simulink model "main"  (R2021b)
settings: Solver=ode45  StartTime=0.0  StopTime=15  MaxStep=0.0050000000000000001  RelTol=1.0000000000000001e-09  AbsTol=9.9999999999999994e-12
settings Model: Creator=Lenovo  LastModifiedBy=Lenovo
settings DataIOCC: SaveOutput=off  SignalLogging=off  SaveTime=off  OutputOption=SpecifiedOutputTimes  OutputTimes=0:0.005:15

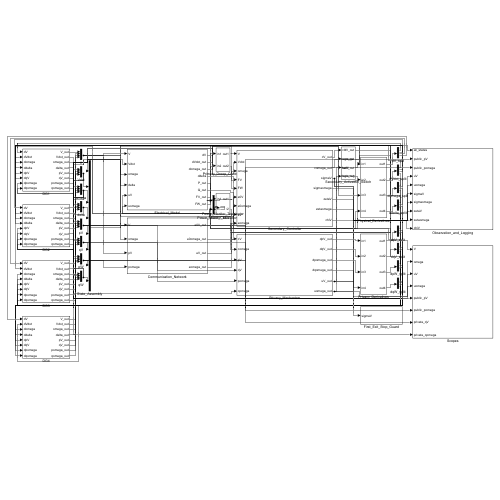
[thumbnail: Simulink's stored preview of the top-level diagram]
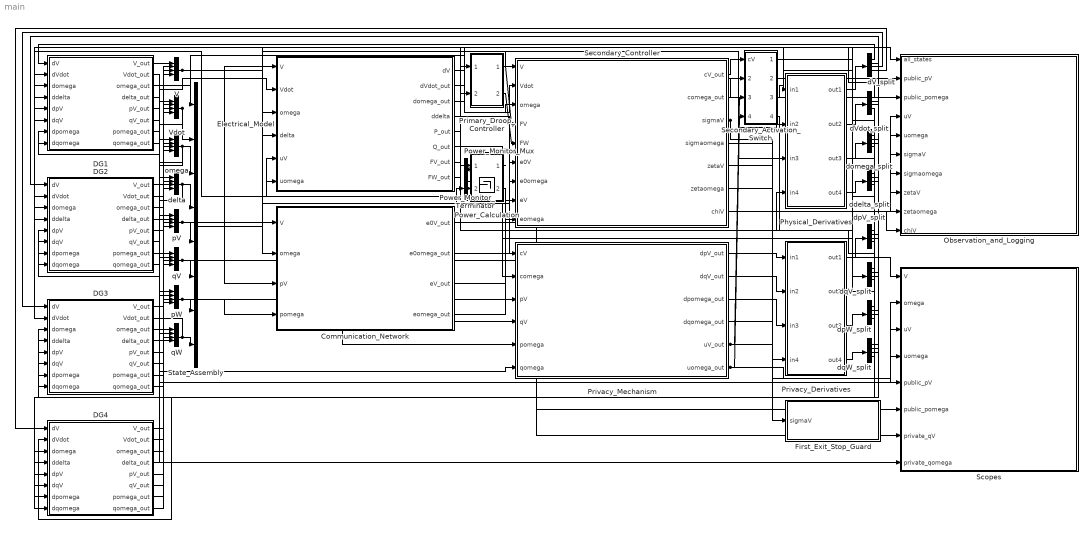
== system main ==
  Communication_Network : Subsystem
  DG1 : Subsystem
  DG2 : Subsystem
  DG3 : Subsystem
  DG4 : Subsystem
  Electrical_Model : Subsystem
  First_Exit_Stop_Guard : Subsystem
  Observation_and_Logging : Subsystem
  Physical_Derivatives : Subsystem
  Power_Calculation : Subsystem
  Power_Monitor_Mux : Mux  Inputs=2
  Power_Monitor_Terminator : Terminator
  Primary_Droop_Controller : Subsystem
  Privacy_Derivatives : Subsystem
  Privacy_Mechanism : Subsystem
  Scopes : Subsystem
  Secondary_Activation_Switch : Subsystem
  Secondary_Controller : Subsystem
  State_Assembly : Mux  Inputs=8
  V : Mux
  Vdot : Mux
  dV_split : Demux
  dVdot_split : Demux
  ddelta_split : Demux
  delta : Mux
  domega_split : Demux
  dpV_split : Demux
  dpW_split : Demux
  dqV_split : Demux
  dqW_split : Demux
  omega : Mux
  pV : Mux
  pW : Mux
  qV : Mux
  qW : Mux
  wires:
  DG1/1(V_out) -> V/1
  DG2/1(V_out) -> V/2
  DG3/1(V_out) -> V/3
  DG4/1(V_out) -> V/4
  V/1 -> State_Assembly/1, Electrical_Model/1(V), Communication_Network/1(V), Secondary_Controller/1(V), Scopes/1(V)
  DG1/2(Vdot_out) -> Vdot/1
  DG2/2(Vdot_out) -> Vdot/2
  DG3/2(Vdot_out) -> Vdot/3
  DG4/2(Vdot_out) -> Vdot/4
  Vdot/1 -> State_Assembly/2, Electrical_Model/2(Vdot), Secondary_Controller/2(Vdot)
  DG1/3(omega_out) -> omega/1
  DG2/3(omega_out) -> omega/2
  DG3/3(omega_out) -> omega/3
  DG4/3(omega_out) -> omega/4
  omega/1 -> State_Assembly/3, Electrical_Model/3(omega), Communication_Network/2(omega), Secondary_Controller/3(omega), Scopes/2(omega)
  DG1/4(delta_out) -> delta/1
  DG2/4(delta_out) -> delta/2
  DG3/4(delta_out) -> delta/3
  DG4/4(delta_out) -> delta/4
  delta/1 -> State_Assembly/4, Electrical_Model/4(delta)
  DG1/5(pV_out) -> pV/1
  DG2/5(pV_out) -> pV/2
  DG3/5(pV_out) -> pV/3
  DG4/5(pV_out) -> pV/4
  pV/1 -> State_Assembly/5, Communication_Network/3(pV), Privacy_Mechanism/3(pV), Observation_and_Logging/2(public_pV), Scopes/5(public_pV)
  DG1/6(qV_out) -> qV/1
  DG2/6(qV_out) -> qV/2
  DG3/6(qV_out) -> qV/3
  DG4/6(qV_out) -> qV/4
  qV/1 -> State_Assembly/6, Privacy_Mechanism/4(qV), Scopes/7(private_qV)
  DG1/7(pomega_out) -> pW/1
  DG2/7(pomega_out) -> pW/2
  DG3/7(pomega_out) -> pW/3
  DG4/7(pomega_out) -> pW/4
  pW/1 -> State_Assembly/7, Communication_Network/4(pomega), Privacy_Mechanism/5(pomega), Observation_and_Logging/3(public_pomega), Scopes/6(public_pomega)
  DG1/8(qomega_out) -> qW/1
  DG2/8(qomega_out) -> qW/2
  DG3/8(qomega_out) -> qW/3
  DG4/8(qomega_out) -> qW/4
  qW/1 -> State_Assembly/8, Privacy_Mechanism/6(qomega), Scopes/8(private_qomega)
  Secondary_Activation_Switch/3(hatV_out) -> Electrical_Model/5(uV)
  Secondary_Activation_Switch/4(hatomega_out) -> Electrical_Model/6(uomega)
  Electrical_Model/1(dV) -> Physical_Derivatives/1(in1)
  Electrical_Model/2(dVdot_out) -> Physical_Derivatives/2(in2)
  Electrical_Model/3(domega_out) -> Physical_Derivatives/3(in3)
  Electrical_Model/4(ddelta) -> Physical_Derivatives/4(in4)
  Electrical_Model/7(FV_out) -> Primary_Droop_Controller/1(in1)
  Electrical_Model/8(FW_out) -> Primary_Droop_Controller/2(in2)
  Primary_Droop_Controller/1(out1) -> Secondary_Controller/4(FV)
  Primary_Droop_Controller/2(out2) -> Secondary_Controller/5(FW)
  Electrical_Model/5(P_out) -> Power_Calculation/1(in1)
  Electrical_Model/6(Q_out) -> Power_Calculation/2(in2)
  Power_Calculation/1(out1) -> Power_Monitor_Mux/1
  Power_Calculation/2(out2) -> Power_Monitor_Mux/2
  Power_Monitor_Mux/1 -> Power_Monitor_Terminator/1
  Communication_Network/1(e0V_out) -> Secondary_Controller/6(e0V)
  Communication_Network/2(e0omega_out) -> Secondary_Controller/7(e0omega)
  Communication_Network/3(eV_out) -> Secondary_Controller/8(eV)
  Communication_Network/4(eomega_out) -> Secondary_Controller/9(eomega)
  Secondary_Controller/1(cV_out) -> Secondary_Activation_Switch/1(cV)
  Secondary_Controller/2(comega_out) -> Secondary_Activation_Switch/2(comega)
  Secondary_Activation_Switch/1(cV_out) -> Privacy_Mechanism/1(cV)
  Secondary_Activation_Switch/2(comega_out) -> Privacy_Mechanism/2(comega)
  Privacy_Mechanism/5(uV_out) -> Secondary_Activation_Switch/3(hatV), Observation_and_Logging/4(uV), Scopes/3(uV)
  Privacy_Mechanism/6(uomega_out) -> Secondary_Activation_Switch/4(hatomega), Observation_and_Logging/5(uomega), Scopes/4(uomega)
  Privacy_Mechanism/1(dpV_out) -> Privacy_Derivatives/1(in1)
  Privacy_Mechanism/2(dqV_out) -> Privacy_Derivatives/2(in2)
  Privacy_Mechanism/3(dpomega_out) -> Privacy_Derivatives/3(in3)
  Privacy_Mechanism/4(dqomega_out) -> Privacy_Derivatives/4(in4)
  Physical_Derivatives/1(out1) -> dV_split/1
  dV_split/1 -> DG1/1(dV)
  dV_split/2 -> DG2/1(dV)
  dV_split/3 -> DG3/1(dV)
  dV_split/4 -> DG4/1(dV)
  Physical_Derivatives/2(out2) -> dVdot_split/1
  dVdot_split/1 -> DG1/2(dVdot)
  dVdot_split/2 -> DG2/2(dVdot)
  dVdot_split/3 -> DG3/2(dVdot)
  dVdot_split/4 -> DG4/2(dVdot)
  Physical_Derivatives/3(out3) -> domega_split/1
  domega_split/1 -> DG1/3(domega)
  domega_split/2 -> DG2/3(domega)
  domega_split/3 -> DG3/3(domega)
  domega_split/4 -> DG4/3(domega)
  Physical_Derivatives/4(out4) -> ddelta_split/1
  ddelta_split/1 -> DG1/4(ddelta)
  ddelta_split/2 -> DG2/4(ddelta)
  ddelta_split/3 -> DG3/4(ddelta)
  ddelta_split/4 -> DG4/4(ddelta)
  Privacy_Derivatives/1(out1) -> dpV_split/1
  dpV_split/1 -> DG1/5(dpV)
  dpV_split/2 -> DG2/5(dpV)
  dpV_split/3 -> DG3/5(dpV)
  dpV_split/4 -> DG4/5(dpV)
  Privacy_Derivatives/2(out2) -> dqV_split/1
  dqV_split/1 -> DG1/6(dqV)
  dqV_split/2 -> DG2/6(dqV)
  dqV_split/3 -> DG3/6(dqV)
  dqV_split/4 -> DG4/6(dqV)
  Privacy_Derivatives/3(out3) -> dpW_split/1
  dpW_split/1 -> DG1/7(dpomega)
  dpW_split/2 -> DG2/7(dpomega)
  dpW_split/3 -> DG3/7(dpomega)
  dpW_split/4 -> DG4/7(dpomega)
  Privacy_Derivatives/4(out4) -> dqW_split/1
  dqW_split/1 -> DG1/8(dqomega)
  dqW_split/2 -> DG2/8(dqomega)
  dqW_split/3 -> DG3/8(dqomega)
  dqW_split/4 -> DG4/8(dqomega)
  State_Assembly/1 -> Observation_and_Logging/1(all_states)
  Secondary_Controller/3(sigmaV) -> Observation_and_Logging/6(sigmaV), First_Exit_Stop_Guard/1(sigmaV)
  Secondary_Controller/4(sigmaomega) -> Observation_and_Logging/7(sigmaomega)
  Secondary_Controller/5(zetaV) -> Observation_and_Logging/8(zetaV)
  Secondary_Controller/6(zetaomega) -> Observation_and_Logging/9(zetaomega)
  Secondary_Controller/7(chiV) -> Observation_and_Logging/10(chiV)

== system main/Communication_Network ==
  V : Inport
  omega : Inport  Port=2
  pV : Inport  Port=3
  pomega : Inport  Port=4
  LpV : Gain  Gain=[1 -1 0 0;-1 2 -1 0;0 -1 2 -1;0 0 -1 1]  Multiplication=Matrix(K*u)
  LpW : Gain  Gain=[1 -1 0 0;-1 2 -1 0;0 -1 2 -1;0 0 -1 1]  Multiplication=Matrix(K*u)
  e0V : Bias  Bias=-1
  e0V_Gain : Gain  Gain=[1 0 0 0;0 1 0 0;0 0 1 0;0 0 0 1]  Multiplication=Matrix(K*u)
  e0omega : Bias
  e0omega_Gain : Gain  Gain=[1 0 0 0;0 1 0 0;0 0 1 0;0 0 0 1]  Multiplication=Matrix(K*u)
  eV : Sum
  eW : Sum
  pinV : Gain  Gain=[1 0 0 0;0 0 0 0;0 0 0 0;0 0 0 0]  Multiplication=Matrix(K*u)
  pinW : Gain  Gain=[1 0 0 0;0 0 0 0;0 0 0 0;0 0 0 0]  Multiplication=Matrix(K*u)
  e0V_out : Outport
  e0omega_out : Outport  Port=2
  eV_out : Outport  Port=3
  eomega_out : Outport  Port=4
  wires:
  V/1 -> e0V/1
  e0V/1 -> e0V_Gain/1
  omega/1 -> e0omega/1
  e0omega/1 -> e0omega_Gain/1
  e0V_Gain/1 -> pinV/1, e0V_out/1
  pV/1 -> LpV/1
  e0omega_Gain/1 -> pinW/1, e0omega_out/1
  pomega/1 -> LpW/1
  pinV/1 -> eV/1
  LpV/1 -> eV/2
  pinW/1 -> eW/1
  LpW/1 -> eW/2
  eV/1 -> eV_out/1
  eW/1 -> eomega_out/1

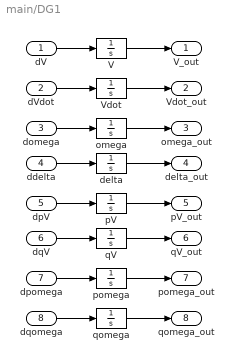
== system main/DG1 ==
  dV : Inport
  dVdot : Inport  Port=2
  domega : Inport  Port=3
  ddelta : Inport  Port=4
  dpV : Inport  Port=5
  dqV : Inport  Port=6
  dpomega : Inport  Port=7
  dqomega : Inport  Port=8
  V : Integrator  InitialCondition=1.0012000000000001
  Vdot : Integrator
  delta : Integrator  InitialCondition=0.01
  omega : Integrator  InitialCondition=0.00069999999999999999
  pV : Integrator  InitialCondition=0.01
  pomega : Integrator  InitialCondition=0.0080000000000000002
  qV : Integrator  InitialCondition=-0.01
  qomega : Integrator  InitialCondition=-0.0080000000000000002
  V_out : Outport
  Vdot_out : Outport  Port=2
  omega_out : Outport  Port=3
  delta_out : Outport  Port=4
  pV_out : Outport  Port=5
  qV_out : Outport  Port=6
  pomega_out : Outport  Port=7
  qomega_out : Outport  Port=8
  wires:
  dV/1 -> V/1
  V/1 -> V_out/1
  dVdot/1 -> Vdot/1
  Vdot/1 -> Vdot_out/1
  domega/1 -> omega/1
  omega/1 -> omega_out/1
  ddelta/1 -> delta/1
  delta/1 -> delta_out/1
  dpV/1 -> pV/1
  pV/1 -> pV_out/1
  dqV/1 -> qV/1
  qV/1 -> qV_out/1
  dpomega/1 -> pomega/1
  pomega/1 -> pomega_out/1
  dqomega/1 -> qomega/1
  qomega/1 -> qomega_out/1

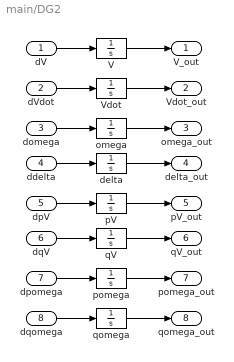
== system main/DG2 ==
  dV : Inport
  dVdot : Inport  Port=2
  domega : Inport  Port=3
  ddelta : Inport  Port=4
  dpV : Inport  Port=5
  dqV : Inport  Port=6
  dpomega : Inport  Port=7
  dqomega : Inport  Port=8
  V : Integrator  InitialCondition=1.0009999999999999
  Vdot : Integrator
  delta : Integrator  InitialCondition=0.0050000000000000001
  omega : Integrator  InitialCondition=0.00050000000000000001
  pV : Integrator  InitialCondition=-0.0080000000000000002
  pomega : Integrator  InitialCondition=-0.0060000000000000001
  qV : Integrator  InitialCondition=0.0080000000000000002
  qomega : Integrator  InitialCondition=0.0060000000000000001
  V_out : Outport
  Vdot_out : Outport  Port=2
  omega_out : Outport  Port=3
  delta_out : Outport  Port=4
  pV_out : Outport  Port=5
  qV_out : Outport  Port=6
  pomega_out : Outport  Port=7
  qomega_out : Outport  Port=8
  wires:
  dV/1 -> V/1
  V/1 -> V_out/1
  dVdot/1 -> Vdot/1
  Vdot/1 -> Vdot_out/1
  domega/1 -> omega/1
  omega/1 -> omega_out/1
  ddelta/1 -> delta/1
  delta/1 -> delta_out/1
  dpV/1 -> pV/1
  pV/1 -> pV_out/1
  dqV/1 -> qV/1
  qV/1 -> qV_out/1
  dpomega/1 -> pomega/1
  pomega/1 -> pomega_out/1
  dqomega/1 -> qomega/1
  qomega/1 -> qomega_out/1

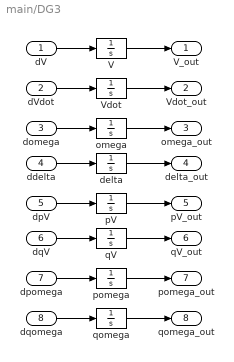
== system main/DG3 ==
  dV : Inport
  dVdot : Inport  Port=2
  domega : Inport  Port=3
  ddelta : Inport  Port=4
  dpV : Inport  Port=5
  dqV : Inport  Port=6
  dpomega : Inport  Port=7
  dqomega : Inport  Port=8
  V : Integrator  InitialCondition=1.0007999999999999
  Vdot : Integrator
  delta : Integrator  InitialCondition=-0.0030000000000000001
  omega : Integrator  InitialCondition=0.00040000000000000002
  pV : Integrator  InitialCondition=0.0060000000000000001
  pomega : Integrator  InitialCondition=0.0050000000000000001
  qV : Integrator  InitialCondition=-0.0060000000000000001
  qomega : Integrator  InitialCondition=-0.0050000000000000001
  V_out : Outport
  Vdot_out : Outport  Port=2
  omega_out : Outport  Port=3
  delta_out : Outport  Port=4
  pV_out : Outport  Port=5
  qV_out : Outport  Port=6
  pomega_out : Outport  Port=7
  qomega_out : Outport  Port=8
  wires:
  dV/1 -> V/1
  V/1 -> V_out/1
  dVdot/1 -> Vdot/1
  Vdot/1 -> Vdot_out/1
  domega/1 -> omega/1
  omega/1 -> omega_out/1
  ddelta/1 -> delta/1
  delta/1 -> delta_out/1
  dpV/1 -> pV/1
  pV/1 -> pV_out/1
  dqV/1 -> qV/1
  qV/1 -> qV_out/1
  dpomega/1 -> pomega/1
  pomega/1 -> pomega_out/1
  dqomega/1 -> qomega/1
  qomega/1 -> qomega_out/1

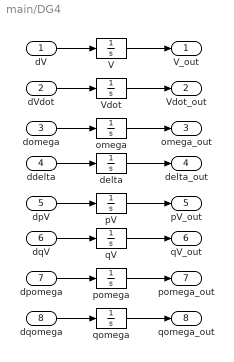
== system main/DG4 ==
  dV : Inport
  dVdot : Inport  Port=2
  domega : Inport  Port=3
  ddelta : Inport  Port=4
  dpV : Inport  Port=5
  dqV : Inport  Port=6
  dpomega : Inport  Port=7
  dqomega : Inport  Port=8
  V : Integrator  InitialCondition=1.0011000000000001
  Vdot : Integrator
  delta : Integrator  InitialCondition=-0.0080000000000000002
  omega : Integrator  InitialCondition=0.00059999999999999995
  pV : Integrator  InitialCondition=-0.0050000000000000001
  pomega : Integrator  InitialCondition=-0.0040000000000000001
  qV : Integrator  InitialCondition=0.0050000000000000001
  qomega : Integrator  InitialCondition=0.0040000000000000001
  V_out : Outport
  Vdot_out : Outport  Port=2
  omega_out : Outport  Port=3
  delta_out : Outport  Port=4
  pV_out : Outport  Port=5
  qV_out : Outport  Port=6
  pomega_out : Outport  Port=7
  qomega_out : Outport  Port=8
  wires:
  dV/1 -> V/1
  V/1 -> V_out/1
  dVdot/1 -> Vdot/1
  Vdot/1 -> Vdot_out/1
  domega/1 -> omega/1
  omega/1 -> omega_out/1
  ddelta/1 -> delta/1
  delta/1 -> delta_out/1
  dpV/1 -> pV/1
  pV/1 -> pV_out/1
  dqV/1 -> qV/1
  qV/1 -> qV_out/1
  dpomega/1 -> pomega/1
  pomega/1 -> pomega_out/1
  dqomega/1 -> qomega/1
  qomega/1 -> qomega_out/1

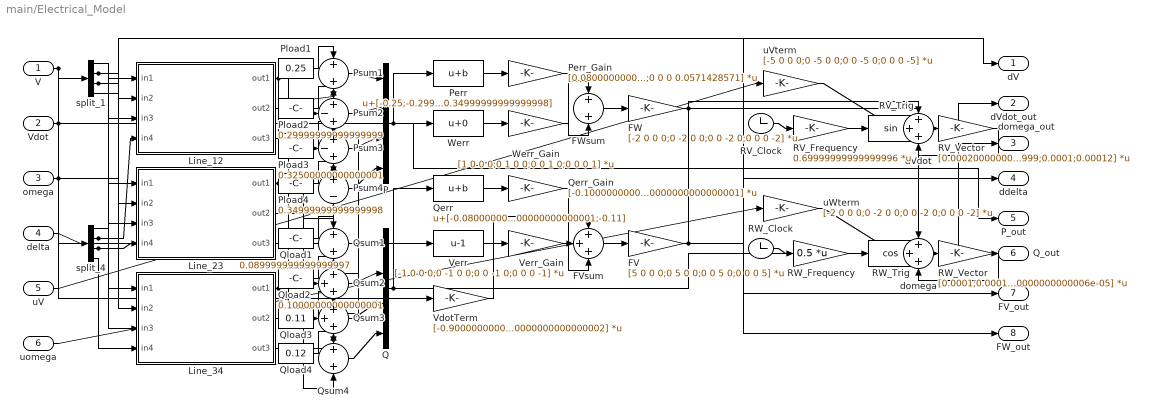
== system main/Electrical_Model ==
  V : Inport
  Vdot : Inport  Port=2
  omega : Inport  Port=3
  delta : Inport  Port=4
  uV : Inport  Port=5
  uomega : Inport  Port=6
  FV : Gain  Gain=[5 0 0 0;0 5 0 0;0 0 5 0;0 0 0 5]  Multiplication=Matrix(K*u)
  FVsum : Sum  Inputs=+++
  FW : Gain  Gain=[-2 0 0 0;0 -2 0 0;0 0 -2 0;0 0 0 -2]  Multiplication=Matrix(K*u)
  FWsum : Sum
  Line_12 : Subsystem
  Line_23 : Subsystem
  Line_34 : Subsystem
  P : Mux
  Perr : Bias  Bias=[-0.25;-0.29999999999999999;-0.32500000000000001;-0.34999999999999998]
  Perr_Gain : Gain  Gain=[0.080000000000000002 0 0 0;0 0.066666666700000002 0 0;0 0 0.061538461500000002 0;0 0 0 0.0571428571]  Multiplication=Matrix(K*u)
  Pload1 : Constant  Value=0.25
  Pload2 : Constant  Value=0.29999999999999999
  Pload3 : Constant  Value=0.32500000000000001
  Pload4 : Constant  Value=0.34999999999999998
  Psum1 : Sum
  Psum2 : Sum  Inputs=+-+
  Psum3 : Sum  Inputs=+-+
  Psum4 : Sum  Inputs=+-
  Q : Mux
  Qerr : Bias  Bias=[-0.080000000000000002;-0.089999999999999997;-0.10000000000000001;-0.11]
  Qerr_Gain : Gain  Gain=[-0.10000000000000001 0 0 0;0 -0.10000000000000001 0 0;0 0 -0.10000000000000001 0;0 0 0 -0.10000000000000001]  Multiplication=Matrix(K*u)
  Qload1 : Constant  Value=0.089999999999999997
  Qload2 : Constant  Value=0.10000000000000001
  Qload3 : Constant  Value=0.11
  Qload4 : Constant  Value=0.12
  Qsum1 : Sum
  Qsum2 : Sum  Inputs=+++
  Qsum3 : Sum  Inputs=+++
  Qsum4 : Sum
  RV_Clock : Clock
  RV_Frequency : Gain  Gain=0.69999999999999996  Multiplication=Matrix(K*u)
  RV_Trig : Trigonometry
  RV_Vector : Gain  Gain=[0.00020000000000000001;0.00014999999999999999;0.0001;0.00012]  Multiplication=Matrix(K*u)
  RW_Clock : Clock
  RW_Frequency : Gain  Gain=0.5  Multiplication=Matrix(K*u)
  RW_Trig : Trigonometry  Operator=cos
  RW_Vector : Gain  Gain=[0.0001;0.00012;8.0000000000000007e-05;9.0000000000000006e-05]  Multiplication=Matrix(K*u)
  VdotTerm : Gain  Gain=[-0.90000000000000002 0 0 0;0 -0.90000000000000002 0 0;0 0 -0.90000000000000002 0;0 0 0 -0.90000000000000002]  Multiplication=Matrix(K*u)
  Verr : Bias  Bias=-1
  Verr_Gain : Gain  Gain=[-1 0 0 0;0 -1 0 0;0 0 -1 0;0 0 0 -1]  Multiplication=Matrix(K*u)
  Werr : Bias
  Werr_Gain : Gain  Gain=[1 0 0 0;0 1 0 0;0 0 1 0;0 0 0 1]  Multiplication=Matrix(K*u)
  dVdot : Sum  Inputs=+++
  domega : Sum  Inputs=+++
  split_1 : Demux
  split_4 : Demux
  uVterm : Gain  Gain=[-5 0 0 0;0 -5 0 0;0 0 -5 0;0 0 0 -5]  Multiplication=Matrix(K*u)
  uWterm : Gain  Gain=[-2 0 0 0;0 -2 0 0;0 0 -2 0;0 0 0 -2]  Multiplication=Matrix(K*u)
  dV : Outport
  dVdot_out : Outport  Port=2
  domega_out : Outport  Port=3
  ddelta : Outport  Port=4
  P_out : Outport  Port=5
  Q_out : Outport  Port=6
  FV_out : Outport  Port=7
  FW_out : Outport  Port=8
  wires:
  V/1 -> split_1/1, Verr/1
  delta/1 -> split_4/1
  split_1/1 -> Line_12/1(in1)
  split_4/1 -> Line_12/3(in3)
  split_1/2 -> Line_12/2(in2), Line_23/1(in1)
  split_4/2 -> Line_12/4(in4), Line_23/3(in3)
  split_1/3 -> Line_23/2(in2), Line_34/1(in1)
  split_4/3 -> Line_23/4(in4), Line_34/3(in3)
  split_1/4 -> Line_34/2(in2)
  split_4/4 -> Line_34/4(in4)
  Pload1/1 -> Psum1/1
  Qload1/1 -> Qsum1/1
  Line_12/1(out1) -> Psum1/2, Psum2/2
  Line_12/2(out2) -> Qsum1/2
  Pload2/1 -> Psum2/1
  Qload2/1 -> Qsum2/1
  Line_12/3(out3) -> Qsum2/2
  Line_23/1(out1) -> Psum2/3, Psum3/2
  Line_23/2(out2) -> Qsum2/3
  Pload3/1 -> Psum3/1
  Qload3/1 -> Qsum3/1
  Line_23/3(out3) -> Qsum3/2
  Line_34/1(out1) -> Psum3/3, Psum4/2
  Line_34/2(out2) -> Qsum3/3
  Pload4/1 -> Psum4/1
  Qload4/1 -> Qsum4/1
  Line_34/3(out3) -> Qsum4/2
  Psum1/1 -> P/1
  Qsum1/1 -> Q/1
  Psum2/1 -> P/2
  Qsum2/1 -> Q/2
  Psum3/1 -> P/3
  Qsum3/1 -> Q/3
  Psum4/1 -> P/4
  Qsum4/1 -> Q/4
  P/1 -> Perr/1, P_out/1
  Perr/1 -> Perr_Gain/1
  omega/1 -> Werr/1, ddelta/1
  Werr/1 -> Werr_Gain/1
  Werr_Gain/1 -> FWsum/1
  Perr_Gain/1 -> FWsum/2
  FWsum/1 -> FW/1
  Q/1 -> Qerr/1, Q_out/1
  Qerr/1 -> Qerr_Gain/1
  Verr/1 -> Verr_Gain/1
  Vdot/1 -> VdotTerm/1, dV/1
  VdotTerm/1 -> FVsum/1
  Verr_Gain/1 -> FVsum/2
  Qerr_Gain/1 -> FVsum/3
  FVsum/1 -> FV/1
  uV/1 -> uVterm/1
  uomega/1 -> uWterm/1
  RV_Clock/1 -> RV_Frequency/1
  RV_Frequency/1 -> RV_Trig/1
  RV_Trig/1 -> RV_Vector/1
  RW_Clock/1 -> RW_Frequency/1
  RW_Frequency/1 -> RW_Trig/1
  RW_Trig/1 -> RW_Vector/1
  FV/1 -> dVdot/1, FV_out/1
  uVterm/1 -> dVdot/2
  RV_Vector/1 -> dVdot/3
  FW/1 -> domega/1, FW_out/1
  uWterm/1 -> domega/2
  RW_Vector/1 -> domega/3
  dVdot/1 -> dVdot_out/1
  domega/1 -> domega_out/1

== system main/First_Exit_Stop_Guard ==
  sigmaV : Inport
  AtOrBeyondBoundary : RelationalOperator  OutDataTypeStr=boolean  RndMeth=Simplest
  BoundaryCount : Gain  Gain=[1 1 1 1]  Multiplication=Matrix(K*u)
  BoundaryDouble : DataTypeConversion  OutDataTypeStr=double
  FunnelBoundary : Constant  Value=[0.99999998999999995;0.99999998999999995;0.99999998999999995;0.99999998999999995]
  StopAtFirstExit : Stop
  abs_sigmaV : Abs
  wires:
  sigmaV/1 -> abs_sigmaV/1
  abs_sigmaV/1 -> AtOrBeyondBoundary/1
  FunnelBoundary/1 -> AtOrBeyondBoundary/2
  AtOrBeyondBoundary/1 -> BoundaryDouble/1
  BoundaryDouble/1 -> BoundaryCount/1
  BoundaryCount/1 -> StopAtFirstExit/1

== system main/Observation_and_Logging ==
  all_states : Inport
  public_pV : Inport  Port=2
  public_pomega : Inport  Port=3
  uV : Inport  Port=4
  uomega : Inport  Port=5
  sigmaV : Inport  Port=6
  sigmaomega : Inport  Port=7
  zetaV : Inport  Port=8
  zetaomega : Inport  Port=9
  chiV : Inport  Port=10
  Control_Inputs : Mux  Inputs=2
  Control_Log : ToWorkspace  VariableName=sim_control  SaveFormat=Structure With Time  SampleTime=-1
  Diagnostic_Log : ToWorkspace  VariableName=sim_diagnostics  SaveFormat=Structure With Time  SampleTime=-1
  Internal_Diagnostics : Mux  Inputs=5
  Public_History : Mux  Inputs=2
  Public_Log : ToWorkspace  VariableName=sim_public  SaveFormat=Structure With Time  SampleTime=-1
  State_Log : ToWorkspace  VariableName=sim_state  SaveFormat=Structure With Time  SampleTime=-1
  wires:
  all_states/1 -> State_Log/1
  public_pV/1 -> Public_History/1
  public_pomega/1 -> Public_History/2
  Public_History/1 -> Public_Log/1
  uV/1 -> Control_Inputs/1
  uomega/1 -> Control_Inputs/2
  Control_Inputs/1 -> Control_Log/1
  sigmaV/1 -> Internal_Diagnostics/1
  sigmaomega/1 -> Internal_Diagnostics/2
  zetaV/1 -> Internal_Diagnostics/3
  zetaomega/1 -> Internal_Diagnostics/4
  chiV/1 -> Internal_Diagnostics/5
  Internal_Diagnostics/1 -> Diagnostic_Log/1

== system main/Physical_Derivatives ==
  in1 : Inport
  in2 : Inport  Port=2
  in3 : Inport  Port=3
  in4 : Inport  Port=4
  out1 : Outport
  out2 : Outport  Port=2
  out3 : Outport  Port=3
  out4 : Outport  Port=4
  wires:
  in1/1 -> out1/1
  in2/1 -> out2/1
  in3/1 -> out3/1
  in4/1 -> out4/1

== system main/Power_Calculation ==
  in1 : Inport
  in2 : Inport  Port=2
  out1 : Outport
  out2 : Outport  Port=2
  wires:
  in1/1 -> out1/1
  in2/1 -> out2/1

== system main/Primary_Droop_Controller ==
  in1 : Inport
  in2 : Inport  Port=2
  out1 : Outport
  out2 : Outport  Port=2
  wires:
  in1/1 -> out1/1
  in2/1 -> out2/1

== system main/Privacy_Derivatives ==
  in1 : Inport
  in2 : Inport  Port=2
  in3 : Inport  Port=3
  in4 : Inport  Port=4
  out1 : Outport
  out2 : Outport  Port=2
  out3 : Outport  Port=3
  out4 : Outport  Port=4
  wires:
  in1/1 -> out1/1
  in2/1 -> out2/1
  in3/1 -> out3/1
  in4/1 -> out4/1

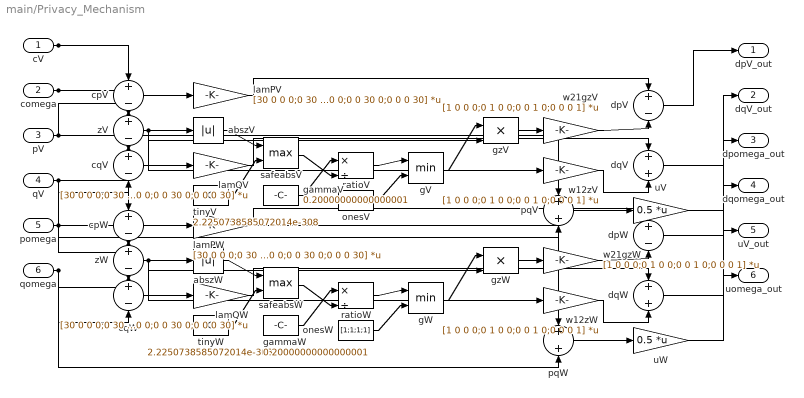
== system main/Privacy_Mechanism ==
  cV : Inport
  comega : Inport  Port=2
  pV : Inport  Port=3
  qV : Inport  Port=4
  pomega : Inport  Port=5
  qomega : Inport  Port=6
  abszV : Abs
  abszW : Abs
  cpV : Sum  Inputs=+-
  cpW : Sum  Inputs=+-
  cqV : Sum  Inputs=+-
  cqW : Sum  Inputs=+-
  dpV : Sum  Inputs=+-
  dpW : Sum  Inputs=+-
  dqV : Sum
  dqW : Sum
  gV : MinMax  Inputs=2
  gW : MinMax  Inputs=2
  gammaV : Constant  Value=0.20000000000000001
  gammaW : Constant  Value=0.20000000000000001
  gzV : Product  Inputs=**
  gzW : Product  Inputs=**
  lamPV : Gain  Gain=[30 0 0 0;0 30 0 0;0 0 30 0;0 0 0 30]  Multiplication=Matrix(K*u)
  lamPW : Gain  Gain=[30 0 0 0;0 30 0 0;0 0 30 0;0 0 0 30]  Multiplication=Matrix(K*u)
  lamQV : Gain  Gain=[30 0 0 0;0 30 0 0;0 0 30 0;0 0 0 30]  Multiplication=Matrix(K*u)
  lamQW : Gain  Gain=[30 0 0 0;0 30 0 0;0 0 30 0;0 0 0 30]  Multiplication=Matrix(K*u)
  onesV : Constant  Value=[1;1;1;1]
  onesW : Constant  Value=[1;1;1;1]
  pqV : Sum
  pqW : Sum
  ratioV : Product  Inputs=*/
  ratioW : Product  Inputs=*/
  safeabsV : MinMax  Function=max  Inputs=2
  safeabsW : MinMax  Function=max  Inputs=2
  tinyV : Constant  Value=2.2250738585072014e-308
  tinyW : Constant  Value=2.2250738585072014e-308
  uV : Gain  Gain=0.5  Multiplication=Matrix(K*u)
  uW : Gain  Gain=0.5  Multiplication=Matrix(K*u)
  w12zV : Gain  Gain=[1 0 0 0;0 1 0 0;0 0 1 0;0 0 0 1]  Multiplication=Matrix(K*u)
  w12zW : Gain  Gain=[1 0 0 0;0 1 0 0;0 0 1 0;0 0 0 1]  Multiplication=Matrix(K*u)
  w21gzV : Gain  Gain=[1 0 0 0;0 1 0 0;0 0 1 0;0 0 0 1]  Multiplication=Matrix(K*u)
  w21gzW : Gain  Gain=[1 0 0 0;0 1 0 0;0 0 1 0;0 0 0 1]  Multiplication=Matrix(K*u)
  zV : Sum  Inputs=+-
  zW : Sum  Inputs=+-
  dpV_out : Outport
  dqV_out : Outport  Port=2
  dpomega_out : Outport  Port=3
  dqomega_out : Outport  Port=4
  uV_out : Outport  Port=5
  uomega_out : Outport  Port=6
  wires:
  pV/1 -> zV/1, cpV/2, pqV/1
  qV/1 -> zV/2, cqV/2, pqV/2
  cV/1 -> cpV/1, cqV/1
  cpV/1 -> lamPV/1
  cqV/1 -> lamQV/1
  zV/1 -> abszV/1, gzV/2, w12zV/1
  abszV/1 -> safeabsV/1
  tinyV/1 -> safeabsV/2
  gammaV/1 -> ratioV/1
  safeabsV/1 -> ratioV/2
  ratioV/1 -> gV/1
  onesV/1 -> gV/2
  gV/1 -> gzV/1
  gzV/1 -> w21gzV/1
  lamPV/1 -> dpV/1
  w21gzV/1 -> dpV/2
  lamQV/1 -> dqV/1
  w12zV/1 -> dqV/2
  pqV/1 -> uV/1
  pomega/1 -> zW/1, cpW/2, pqW/1
  qomega/1 -> zW/2, cqW/2, pqW/2
  comega/1 -> cpW/1, cqW/1
  cpW/1 -> lamPW/1
  cqW/1 -> lamQW/1
  zW/1 -> abszW/1, gzW/2, w12zW/1
  abszW/1 -> safeabsW/1
  tinyW/1 -> safeabsW/2
  gammaW/1 -> ratioW/1
  safeabsW/1 -> ratioW/2
  ratioW/1 -> gW/1
  onesW/1 -> gW/2
  gW/1 -> gzW/1
  gzW/1 -> w21gzW/1
  lamPW/1 -> dpW/1
  w21gzW/1 -> dpW/2
  lamQW/1 -> dqW/1
  w12zW/1 -> dqW/2
  pqW/1 -> uW/1
  dpV/1 -> dpV_out/1
  dqV/1 -> dqV_out/1
  dpW/1 -> dpomega_out/1
  dqW/1 -> dqomega_out/1
  uV/1 -> uV_out/1
  uW/1 -> uomega_out/1

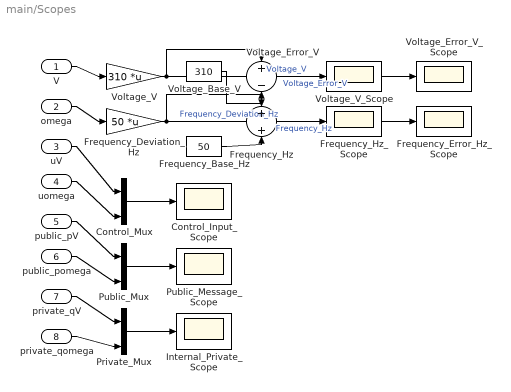
== system main/Scopes ==
  V : Inport
  omega : Inport  Port=2
  uV : Inport  Port=3
  uomega : Inport  Port=4
  public_pV : Inport  Port=5
  public_pomega : Inport  Port=6
  private_qV : Inport  Port=7
  private_qomega : Inport  Port=8
  Control_Input_Scope : Scope
  Control_Mux : Mux  Inputs=2
  Frequency_Base_Hz : Constant  Value=50
  Frequency_Deviation_Hz : Gain  Gain=50  Multiplication=Matrix(K*u)
  Frequency_Error_Hz_Scope : Scope
  Frequency_Hz : Sum
  Frequency_Hz_Scope : Scope
  Internal_Private_Scope : Scope
  Private_Mux : Mux  Inputs=2
  Public_Message_Scope : Scope
  Public_Mux : Mux  Inputs=2
  Voltage_Base_V : Constant  Value=310
  Voltage_Error_V : Sum  Inputs=+-
  Voltage_Error_V_Scope : Scope
  Voltage_V : Gain  Gain=310  Multiplication=Matrix(K*u)
  Voltage_V_Scope : Scope
  wires:
  V/1 -> Voltage_V/1
  omega/1 -> Frequency_Deviation_Hz/1
  Frequency_Deviation_Hz/1 -> Frequency_Hz/1, Frequency_Error_Hz_Scope/1  "Frequency_Deviation_Hz"
  Frequency_Base_Hz/1 -> Frequency_Hz/2
  Voltage_V/1 -> Voltage_Error_V/1, Voltage_V_Scope/1  "Voltage_V"
  Voltage_Base_V/1 -> Voltage_Error_V/2
  Voltage_Error_V/1 -> Voltage_Error_V_Scope/1  "Voltage_Error_V"
  Frequency_Hz/1 -> Frequency_Hz_Scope/1  "Frequency_Hz"
  uV/1 -> Control_Mux/1
  uomega/1 -> Control_Mux/2
  Control_Mux/1 -> Control_Input_Scope/1
  public_pV/1 -> Public_Mux/1
  public_pomega/1 -> Public_Mux/2
  Public_Mux/1 -> Public_Message_Scope/1
  private_qV/1 -> Private_Mux/1
  private_qomega/1 -> Private_Mux/2
  Private_Mux/1 -> Internal_Private_Scope/1

== system main/Secondary_Activation_Switch ==
  cV : Inport
  comega : Inport  Port=2
  hatV : Inport  Port=3
  hatomega : Inport  Port=4
  ActivationTime : Constant  Value=5
  Clock : Clock
  Enabled : RelationalOperator  OutDataTypeStr=boolean  RndMeth=Simplest
  Switch_cV : Switch  Criteria=u2 > Threshold  Threshold=0.5
  Switch_comega : Switch  Criteria=u2 > Threshold  Threshold=0.5
  Switch_hatV : Switch  Criteria=u2 > Threshold  Threshold=0.5
  Switch_hatomega : Switch  Criteria=u2 > Threshold  Threshold=0.5
  ZeroVector : Constant  Value=[0;0;0;0]
  cV_out : Outport
  comega_out : Outport  Port=2
  hatV_out : Outport  Port=3
  hatomega_out : Outport  Port=4
  wires:
  Clock/1 -> Enabled/1
  ActivationTime/1 -> Enabled/2
  cV/1 -> Switch_cV/1
  Enabled/1 -> Switch_cV/2, Switch_comega/2, Switch_hatV/2, Switch_hatomega/2
  ZeroVector/1 -> Switch_cV/3, Switch_comega/3, Switch_hatV/3, Switch_hatomega/3
  Switch_cV/1 -> cV_out/1
  comega/1 -> Switch_comega/1
  Switch_comega/1 -> comega_out/1
  hatV/1 -> Switch_hatV/1
  Switch_hatV/1 -> hatV_out/1
  hatomega/1 -> Switch_hatomega/1
  Switch_hatomega/1 -> hatomega_out/1

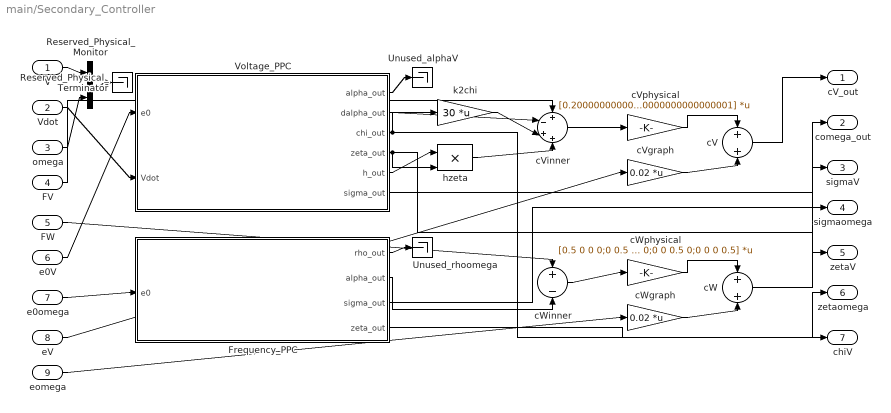
== system main/Secondary_Controller ==
  V : Inport
  Vdot : Inport  Port=2
  omega : Inport  Port=3
  FV : Inport  Port=4
  FW : Inport  Port=5
  e0V : Inport  Port=6
  e0omega : Inport  Port=7
  eV : Inport  Port=8
  eomega : Inport  Port=9
  Frequency_PPC : Subsystem
  Reserved_Physical_Monitor : Mux  Inputs=2
  Reserved_Physical_Terminator : Terminator
  Unused_alphaV : Terminator
  Unused_rhoomega : Terminator
  Voltage_PPC : Subsystem
  cV : Sum
  cVgraph : Gain  Gain=0.02  Multiplication=Matrix(K*u)
  cVinner : Sum  Inputs=+-++
  cVphysical : Gain  Gain=[0.20000000000000001 0 0 0;0 0.20000000000000001 0 0;0 0 0.20000000000000001 0;0 0 0 0.20000000000000001]  Multiplication=Matrix(K*u)
  cW : Sum
  cWgraph : Gain  Gain=0.02  Multiplication=Matrix(K*u)
  cWinner : Sum  Inputs=+-
  cWphysical : Gain  Gain=[0.5 0 0 0;0 0.5 0 0;0 0 0.5 0;0 0 0 0.5]  Multiplication=Matrix(K*u)
  hzeta : Product  Inputs=**
  k2chi : Gain  Gain=30  Multiplication=Matrix(K*u)
  cV_out : Outport
  comega_out : Outport  Port=2
  sigmaV : Outport  Port=3
  sigmaomega : Outport  Port=4
  zetaV : Outport  Port=5
  zetaomega : Outport  Port=6
  chiV : Outport  Port=7
  wires:
  V/1 -> Reserved_Physical_Monitor/1
  omega/1 -> Reserved_Physical_Monitor/2
  Reserved_Physical_Monitor/1 -> Reserved_Physical_Terminator/1
  Voltage_PPC/1(alpha_out) -> Unused_alphaV/1
  Frequency_PPC/1(rho_out) -> Unused_rhoomega/1
  e0V/1 -> Voltage_PPC/1(e0)
  Vdot/1 -> Voltage_PPC/2(Vdot)
  e0omega/1 -> Frequency_PPC/1(e0)
  Voltage_PPC/3(chi_out) -> k2chi/1, chiV/1
  Voltage_PPC/5(h_out) -> hzeta/1
  Voltage_PPC/4(zeta_out) -> hzeta/2, zetaV/1
  FV/1 -> cVinner/1
  Voltage_PPC/2(dalpha_out) -> cVinner/2
  k2chi/1 -> cVinner/3
  hzeta/1 -> cVinner/4
  cVinner/1 -> cVphysical/1
  eV/1 -> cVgraph/1
  cVphysical/1 -> cV/1
  cVgraph/1 -> cV/2
  FW/1 -> cWinner/1
  Frequency_PPC/2(alpha_out) -> cWinner/2
  cWinner/1 -> cWphysical/1
  eomega/1 -> cWgraph/1
  cWphysical/1 -> cW/1
  cWgraph/1 -> cW/2
  cV/1 -> cV_out/1
  cW/1 -> comega_out/1
  Voltage_PPC/6(sigma_out) -> sigmaV/1
  Frequency_PPC/3(sigma_out) -> sigmaomega/1
  Frequency_PPC/4(zeta_out) -> zetaomega/1

== system main/Electrical_Model/Line_12 ==
  in1 : Inport
  in2 : Inport  Port=2
  in3 : Inport  Port=3
  in4 : Inport  Port=4
  Pflow : Gain  Gain=2  Multiplication=Matrix(K*u)
  Praw : Product  Inputs=**
  Q1 : Gain  Gain=2  Multiplication=Matrix(K*u)
  Q1raw : Sum  Inputs=+-
  Q2 : Gain  Gain=2  Multiplication=Matrix(K*u)
  Q2raw : Sum  Inputs=+-
  V1sq : Product  Inputs=**
  V2sq : Product  Inputs=**
  ViVk : Product  Inputs=**
  angle : Sum  Inputs=+-
  cos : Trigonometry  Operator=cos
  crosscos : Product  Inputs=**
  sin : Trigonometry
  out1 : Outport
  out2 : Outport  Port=2
  out3 : Outport  Port=3
  wires:
  in3/1 -> angle/1
  in4/1 -> angle/2
  angle/1 -> sin/1, cos/1
  in1/1 -> ViVk/1, V1sq/1, V1sq/2
  in2/1 -> ViVk/2, V2sq/1, V2sq/2
  ViVk/1 -> Praw/1, crosscos/1
  sin/1 -> Praw/2
  Praw/1 -> Pflow/1
  cos/1 -> crosscos/2
  V1sq/1 -> Q1raw/1
  crosscos/1 -> Q1raw/2, Q2raw/2
  V2sq/1 -> Q2raw/1
  Q1raw/1 -> Q1/1
  Q2raw/1 -> Q2/1
  Pflow/1 -> out1/1
  Q1/1 -> out2/1
  Q2/1 -> out3/1

== system main/Electrical_Model/Line_23 ==
  in1 : Inport
  in2 : Inport  Port=2
  in3 : Inport  Port=3
  in4 : Inport  Port=4
  Pflow : Gain  Gain=1.8  Multiplication=Matrix(K*u)
  Praw : Product  Inputs=**
  Q1 : Gain  Gain=1.8  Multiplication=Matrix(K*u)
  Q1raw : Sum  Inputs=+-
  Q2 : Gain  Gain=1.8  Multiplication=Matrix(K*u)
  Q2raw : Sum  Inputs=+-
  V1sq : Product  Inputs=**
  V2sq : Product  Inputs=**
  ViVk : Product  Inputs=**
  angle : Sum  Inputs=+-
  cos : Trigonometry  Operator=cos
  crosscos : Product  Inputs=**
  sin : Trigonometry
  out1 : Outport
  out2 : Outport  Port=2
  out3 : Outport  Port=3
  wires:
  in3/1 -> angle/1
  in4/1 -> angle/2
  angle/1 -> sin/1, cos/1
  in1/1 -> ViVk/1, V1sq/1, V1sq/2
  in2/1 -> ViVk/2, V2sq/1, V2sq/2
  ViVk/1 -> Praw/1, crosscos/1
  sin/1 -> Praw/2
  Praw/1 -> Pflow/1
  cos/1 -> crosscos/2
  V1sq/1 -> Q1raw/1
  crosscos/1 -> Q1raw/2, Q2raw/2
  V2sq/1 -> Q2raw/1
  Q1raw/1 -> Q1/1
  Q2raw/1 -> Q2/1
  Pflow/1 -> out1/1
  Q1/1 -> out2/1
  Q2/1 -> out3/1

== system main/Electrical_Model/Line_34 ==
  in1 : Inport
  in2 : Inport  Port=2
  in3 : Inport  Port=3
  in4 : Inport  Port=4
  Pflow : Gain  Gain=1.6000000000000001  Multiplication=Matrix(K*u)
  Praw : Product  Inputs=**
  Q1 : Gain  Gain=1.6000000000000001  Multiplication=Matrix(K*u)
  Q1raw : Sum  Inputs=+-
  Q2 : Gain  Gain=1.6000000000000001  Multiplication=Matrix(K*u)
  Q2raw : Sum  Inputs=+-
  V1sq : Product  Inputs=**
  V2sq : Product  Inputs=**
  ViVk : Product  Inputs=**
  angle : Sum  Inputs=+-
  cos : Trigonometry  Operator=cos
  crosscos : Product  Inputs=**
  sin : Trigonometry
  out1 : Outport
  out2 : Outport  Port=2
  out3 : Outport  Port=3
  wires:
  in3/1 -> angle/1
  in4/1 -> angle/2
  angle/1 -> sin/1, cos/1
  in1/1 -> ViVk/1, V1sq/1, V1sq/2
  in2/1 -> ViVk/2, V2sq/1, V2sq/2
  ViVk/1 -> Praw/1, crosscos/1
  sin/1 -> Praw/2
  Praw/1 -> Pflow/1
  cos/1 -> crosscos/2
  V1sq/1 -> Q1raw/1
  crosscos/1 -> Q1raw/2, Q2raw/2
  V2sq/1 -> Q2raw/1
  Q1raw/1 -> Q1/1
  Q2raw/1 -> Q2/1
  Pflow/1 -> out1/1
  Q1/1 -> out2/1
  Q2/1 -> out3/1

== system main/Secondary_Controller/Frequency_PPC ==
  e0 : Inport
  Schedule : Subsystem
  Unused_ddrho : Terminator
  alpha : Sum  Inputs=+-
  k1shapeZeta : Gain  Gain=2  Multiplication=Matrix(K*u)
  oneMinus : Sum  Inputs=+-
  ones : Constant  Value=[1;1;1;1]
  rhoShape : Product  Inputs=**
  shapeZeta : Product  Inputs=**
  sigma : Product  Inputs=*/
  sigma2 : Product  Inputs=**
  stDrho : Product  Inputs=**
  zeta : Trigonometry  Operator=atanh
  rho_out : Outport
  alpha_out : Outport  Port=2
  sigma_out : Outport  Port=3
  zeta_out : Outport  Port=4
  wires:
  Schedule/3(out3) -> Unused_ddrho/1
  e0/1 -> sigma/1
  Schedule/1(out1) -> sigma/2, rhoShape/1, rho_out/1
  sigma/1 -> zeta/1, sigma2/1, sigma2/2, stDrho/1, sigma_out/1
  ones/1 -> oneMinus/1
  sigma2/1 -> oneMinus/2
  oneMinus/1 -> rhoShape/2
  Schedule/2(out2) -> stDrho/2
  rhoShape/1 -> shapeZeta/1
  zeta/1 -> shapeZeta/2, zeta_out/1
  shapeZeta/1 -> k1shapeZeta/1
  stDrho/1 -> alpha/1
  k1shapeZeta/1 -> alpha/2
  alpha/1 -> alpha_out/1

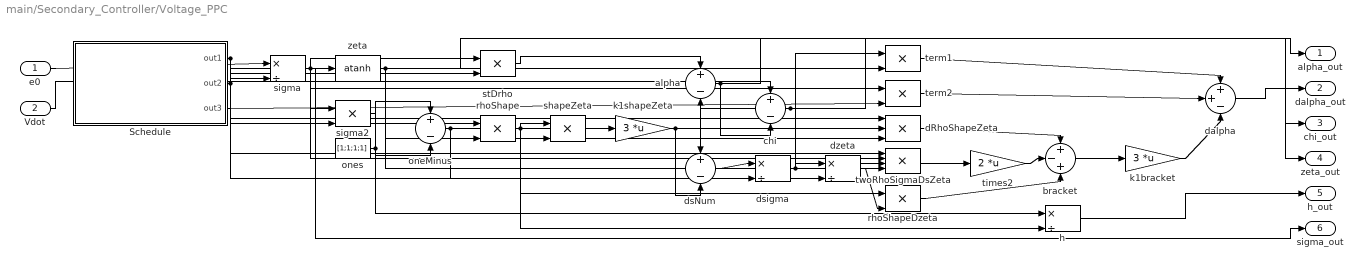
== system main/Secondary_Controller/Voltage_PPC ==
  e0 : Inport
  Vdot : Inport  Port=2
  Schedule : Subsystem
  alpha : Sum  Inputs=+-
  bracket : Sum  Inputs=+-+
  chi : Sum  Inputs=+-
  dRhoShapeZeta : Product  Inputs=***
  dalpha : Sum  Inputs=++-
  dsNum : Sum  Inputs=+-
  dsigma : Product  Inputs=*/
  dzeta : Product  Inputs=*/
  h : Product  Inputs=*/
  k1bracket : Gain  Gain=3  Multiplication=Matrix(K*u)
  k1shapeZeta : Gain  Gain=3  Multiplication=Matrix(K*u)
  oneMinus : Sum  Inputs=+-
  ones : Constant  Value=[1;1;1;1]
  rhoShape : Product  Inputs=**
  rhoShapeDzeta : Product  Inputs=**
  shapeZeta : Product  Inputs=**
  sigma : Product  Inputs=*/
  sigma2 : Product  Inputs=**
  stDrho : Product  Inputs=**
  term1 : Product  Inputs=**
  term2 : Product  Inputs=**
  times2 : Gain  Gain=2  Multiplication=Matrix(K*u)
  twoRhoSigmaDsZeta : Product  Inputs=****
  zeta : Trigonometry  Operator=atanh
  alpha_out : Outport
  dalpha_out : Outport  Port=2
  chi_out : Outport  Port=3
  zeta_out : Outport  Port=4
  h_out : Outport  Port=5
  sigma_out : Outport  Port=6
  wires:
  e0/1 -> sigma/1
  Schedule/1(out1) -> sigma/2, rhoShape/1, dsigma/2, twoRhoSigmaDsZeta/1
  sigma/1 -> zeta/1, sigma2/1, sigma2/2, stDrho/1, term2/1, twoRhoSigmaDsZeta/2, sigma_out/1
  ones/1 -> oneMinus/1, h/1
  sigma2/1 -> oneMinus/2
  oneMinus/1 -> rhoShape/2, dzeta/2, dRhoShapeZeta/2
  Schedule/2(out2) -> stDrho/2, term1/2, dRhoShapeZeta/1
  rhoShape/1 -> shapeZeta/1, rhoShapeDzeta/1, h/2
  zeta/1 -> shapeZeta/2, dRhoShapeZeta/3, twoRhoSigmaDsZeta/4, zeta_out/1
  shapeZeta/1 -> k1shapeZeta/1
  stDrho/1 -> alpha/1
  k1shapeZeta/1 -> alpha/2, dsNum/2
  Vdot/1 -> chi/1
  alpha/1 -> chi/2, alpha_out/1
  chi/1 -> dsNum/1, chi_out/1
  dsNum/1 -> dsigma/1
  dsigma/1 -> dzeta/1, term1/1, twoRhoSigmaDsZeta/3
  Schedule/3(out3) -> term2/2
  twoRhoSigmaDsZeta/1 -> times2/1
  dzeta/1 -> rhoShapeDzeta/2
  dRhoShapeZeta/1 -> bracket/1
  times2/1 -> bracket/2
  rhoShapeDzeta/1 -> bracket/3
  bracket/1 -> k1bracket/1
  term1/1 -> dalpha/1
  term2/1 -> dalpha/2
  k1bracket/1 -> dalpha/3
  dalpha/1 -> dalpha_out/1
  h/1 -> h_out/1

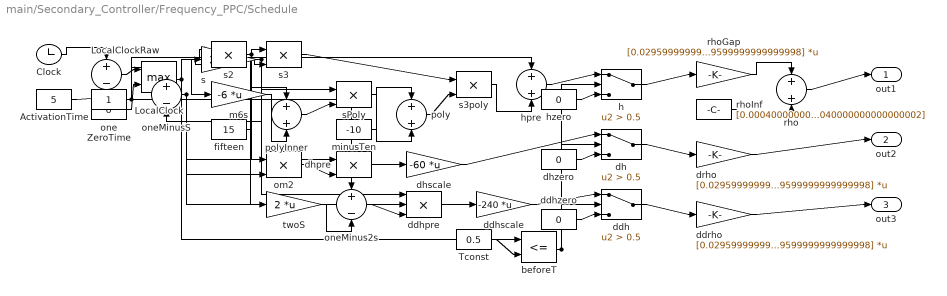
== system main/Secondary_Controller/Frequency_PPC/Schedule ==
  ActivationTime : Constant  Value=5
  Clock : Clock
  LocalClock : MinMax  Function=max  Inputs=2
  LocalClockRaw : Sum  Inputs=+-
  Tconst : Constant  Value=0.5
  ZeroTime : Constant  Value=0
  beforeT : RelationalOperator  Operator=<=  OutDataTypeStr=boolean  RndMeth=Simplest
  ddh : Switch  Criteria=u2 > Threshold  Threshold=0.5
  ddhpre : Product  Inputs=***
  ddhscale : Gain  Gain=-240  Multiplication=Matrix(K*u)
  ddhzero : Constant  Value=0
  ddrho : Gain  Gain=[0.029599999999999998;0.029599999999999998;0.029599999999999998;0.029599999999999998]  Multiplication=Matrix(K*u)
  dh : Switch  Criteria=u2 > Threshold  Threshold=0.5
  dhpre : Product  Inputs=**
  dhscale : Gain  Gain=-60  Multiplication=Matrix(K*u)
  dhzero : Constant  Value=0
  drho : Gain  Gain=[0.029599999999999998;0.029599999999999998;0.029599999999999998;0.029599999999999998]  Multiplication=Matrix(K*u)
  fifteen : Constant  Value=15
  h : Switch  Criteria=u2 > Threshold  Threshold=0.5
  hpre : Sum
  hzero : Constant  Value=0
  m6s : Gain  Gain=-6  Multiplication=Matrix(K*u)
  minusTen : Constant  Value=-10
  om2 : Product  Inputs=**
  one : Constant
  oneMinus2s : Sum  Inputs=+-
  oneMinusS : Sum  Inputs=+-
  poly : Sum
  polyInner : Sum
  rho : Sum
  rhoGap : Gain  Gain=[0.029599999999999998;0.029599999999999998;0.029599999999999998;0.029599999999999998]  Multiplication=Matrix(K*u)
  rhoInf : Constant  Value=[0.00040000000000000002;0.00040000000000000002;0.00040000000000000002;0.00040000000000000002]
  s : Gain  Gain=2  Multiplication=Matrix(K*u)
  s2 : Product  Inputs=**
  s3 : Product  Inputs=**
  s3poly : Product  Inputs=**
  sPoly : Product  Inputs=**
  twoS : Gain  Gain=2  Multiplication=Matrix(K*u)
  out1 : Outport
  out2 : Outport  Port=2
  out3 : Outport  Port=3
  wires:
  Clock/1 -> LocalClockRaw/1
  ActivationTime/1 -> LocalClockRaw/2
  LocalClockRaw/1 -> LocalClock/1
  ZeroTime/1 -> LocalClock/2
  LocalClock/1 -> s/1, beforeT/1
  one/1 -> oneMinusS/1, hpre/1, oneMinus2s/1
  s/1 -> oneMinusS/2, s2/1, s2/2, s3/2, m6s/1, sPoly/1, twoS/1, ddhpre/1
  s2/1 -> s3/1, dhpre/1
  fifteen/1 -> polyInner/1
  m6s/1 -> polyInner/2
  polyInner/1 -> sPoly/2
  minusTen/1 -> poly/1
  sPoly/1 -> poly/2
  s3/1 -> s3poly/1
  poly/1 -> s3poly/2
  s3poly/1 -> hpre/2
  oneMinusS/1 -> om2/1, om2/2, ddhpre/2
  om2/1 -> dhpre/2
  dhpre/1 -> dhscale/1
  twoS/1 -> oneMinus2s/2
  oneMinus2s/1 -> ddhpre/3
  ddhpre/1 -> ddhscale/1
  Tconst/1 -> beforeT/2
  hpre/1 -> h/1
  beforeT/1 -> h/2, dh/2, ddh/2
  hzero/1 -> h/3
  dhscale/1 -> dh/1
  dhzero/1 -> dh/3
  ddhscale/1 -> ddh/1
  ddhzero/1 -> ddh/3
  h/1 -> rhoGap/1
  rhoGap/1 -> rho/1
  rhoInf/1 -> rho/2
  dh/1 -> drho/1
  ddh/1 -> ddrho/1
  rho/1 -> out1/1
  drho/1 -> out2/1
  ddrho/1 -> out3/1

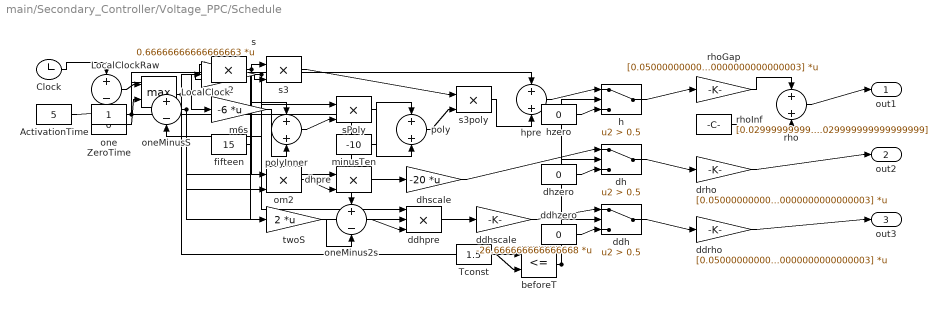
== system main/Secondary_Controller/Voltage_PPC/Schedule ==
  ActivationTime : Constant  Value=5
  Clock : Clock
  LocalClock : MinMax  Function=max  Inputs=2
  LocalClockRaw : Sum  Inputs=+-
  Tconst : Constant  Value=1.5
  ZeroTime : Constant  Value=0
  beforeT : RelationalOperator  Operator=<=  OutDataTypeStr=boolean  RndMeth=Simplest
  ddh : Switch  Criteria=u2 > Threshold  Threshold=0.5
  ddhpre : Product  Inputs=***
  ddhscale : Gain  Gain=-26.666666666666668  Multiplication=Matrix(K*u)
  ddhzero : Constant  Value=0
  ddrho : Gain  Gain=[0.050000000000000003;0.050000000000000003;0.050000000000000003;0.050000000000000003]  Multiplication=Matrix(K*u)
  dh : Switch  Criteria=u2 > Threshold  Threshold=0.5
  dhpre : Product  Inputs=**
  dhscale : Gain  Gain=-20  Multiplication=Matrix(K*u)
  dhzero : Constant  Value=0
  drho : Gain  Gain=[0.050000000000000003;0.050000000000000003;0.050000000000000003;0.050000000000000003]  Multiplication=Matrix(K*u)
  fifteen : Constant  Value=15
  h : Switch  Criteria=u2 > Threshold  Threshold=0.5
  hpre : Sum
  hzero : Constant  Value=0
  m6s : Gain  Gain=-6  Multiplication=Matrix(K*u)
  minusTen : Constant  Value=-10
  om2 : Product  Inputs=**
  one : Constant
  oneMinus2s : Sum  Inputs=+-
  oneMinusS : Sum  Inputs=+-
  poly : Sum
  polyInner : Sum
  rho : Sum
  rhoGap : Gain  Gain=[0.050000000000000003;0.050000000000000003;0.050000000000000003;0.050000000000000003]  Multiplication=Matrix(K*u)
  rhoInf : Constant  Value=[0.029999999999999999;0.029999999999999999;0.029999999999999999;0.029999999999999999]
  s : Gain  Gain=0.66666666666666663  Multiplication=Matrix(K*u)
  s2 : Product  Inputs=**
  s3 : Product  Inputs=**
  s3poly : Product  Inputs=**
  sPoly : Product  Inputs=**
  twoS : Gain  Gain=2  Multiplication=Matrix(K*u)
  out1 : Outport
  out2 : Outport  Port=2
  out3 : Outport  Port=3
  wires:
  Clock/1 -> LocalClockRaw/1
  ActivationTime/1 -> LocalClockRaw/2
  LocalClockRaw/1 -> LocalClock/1
  ZeroTime/1 -> LocalClock/2
  LocalClock/1 -> s/1, beforeT/1
  one/1 -> oneMinusS/1, hpre/1, oneMinus2s/1
  s/1 -> oneMinusS/2, s2/1, s2/2, s3/2, m6s/1, sPoly/1, twoS/1, ddhpre/1
  s2/1 -> s3/1, dhpre/1
  fifteen/1 -> polyInner/1
  m6s/1 -> polyInner/2
  polyInner/1 -> sPoly/2
  minusTen/1 -> poly/1
  sPoly/1 -> poly/2
  s3/1 -> s3poly/1
  poly/1 -> s3poly/2
  s3poly/1 -> hpre/2
  oneMinusS/1 -> om2/1, om2/2, ddhpre/2
  om2/1 -> dhpre/2
  dhpre/1 -> dhscale/1
  twoS/1 -> oneMinus2s/2
  oneMinus2s/1 -> ddhpre/3
  ddhpre/1 -> ddhscale/1
  Tconst/1 -> beforeT/2
  hpre/1 -> h/1
  beforeT/1 -> h/2, dh/2, ddh/2
  hzero/1 -> h/3
  dhscale/1 -> dh/1
  dhzero/1 -> dh/3
  ddhscale/1 -> ddh/1
  ddhzero/1 -> ddh/3
  h/1 -> rhoGap/1
  rhoGap/1 -> rho/1
  rhoInf/1 -> rho/2
  dh/1 -> drho/1
  ddh/1 -> ddrho/1
  rho/1 -> out1/1
  drho/1 -> out2/1
  ddrho/1 -> out3/1
